simulink model "sampleModel1806"  (R2023a)
settings: Solver=VariableStepAuto  StartTime=0.0  StopTime=10.0  RelTol=1e-3
libraries: hdlsllib x4, simulink x1
settings Model: Creator=user1  LastModifiedBy=user1

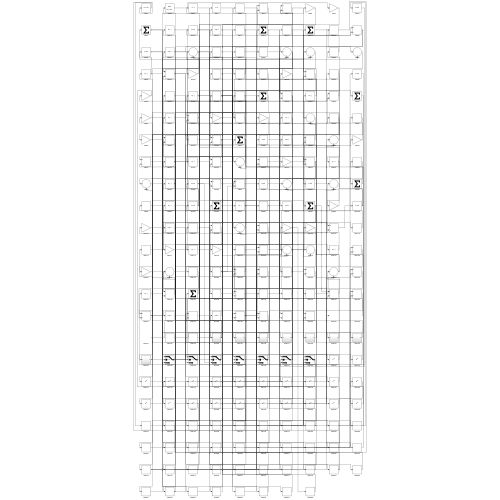
[thumbnail: Simulink's stored preview of the top-level diagram]
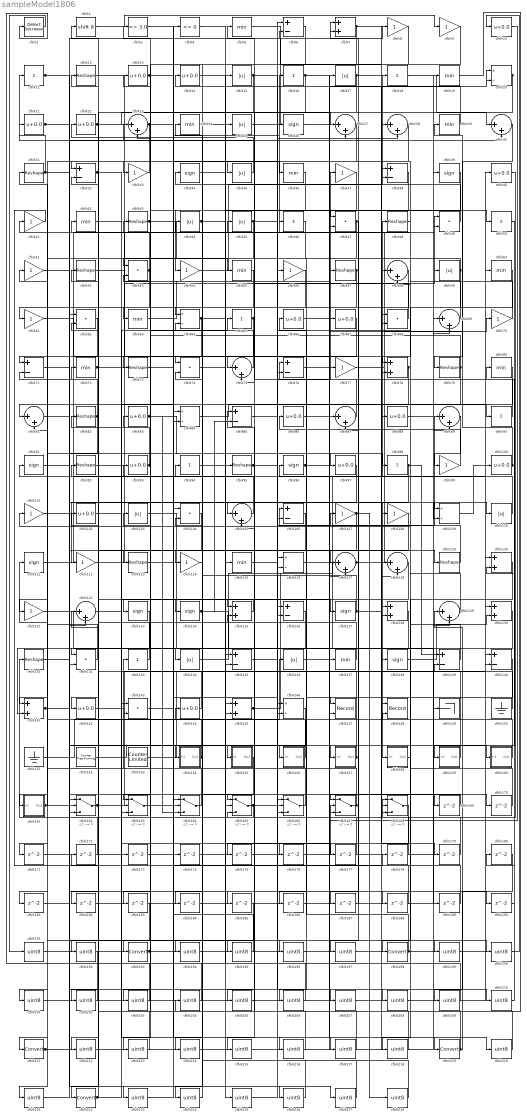
== system sampleModel1806 ==
  cfblk1 : simulink/Logic and Bit Operations/Detect Decrease  vinit=0.0  OutDataTypeStr=boolean
      settings: LibrarySourceBlock=|
      | hdlsllib/Logic and Bit
      | Operations/Detect
      | Decrease
  cfblk{10,13..14,21..22,40,66..67,83,86,88,93,97,100,102,142,144} (17 alike) : Bias  Bias=0.0  SaturateOnIntegerOverflow=off
  cfblk{8..9,33,37,41,51,54,56,61,70,77,99,101,107..108,112,114,121} (18 alike) : Gain
  cfblk{15,17,25,35,44..45,59,103,110,134,136} (11 alike) : Abs  SaturateOnIntegerOverflow=off
  cfblk{47,49,53,62,68,74,104,132,143} (9 alike) : DotProduct  OutDataTypeStr=Inherit: Inherit via internal rule
  cfblk{23,27..28,30,58,69,75,81,87,89,105,117..118,122,129} (15 alike) : Sum  Inputs=|++
  cfblk{6,32,38,71,76,85,106,126,135,139..140} (11 alike) : Sum  Inputs=+-
  cfblk{20,64,84,109,116,146} (6 alike) : Product  Inputs=*/  RndMeth=Zero  SaturateOnIntegerOverflow=on
  cfblk{11,16,18,46,50,65,90,94,98,133} (10 alike) : Sum  Inputs=+
  cfblk{26,34,39,91,96,111,123..124,127,138} (10 alike) : Signum
  cfblk{12,31,43,48,52,57,73,79,82,92,95,113,119,131} (14 alike) : Reshape
  cfblk{5,19,24,29,36,42,55,60,63,72,80,115,137} (13 alike) : MinMax
  cfblk{7,78,120,125,128,130,141,145} (8 alike) : Sum
  cfblk147 : Record  FileSettingsInternal="{\"entries\":[{\"content\":{\"excelSettings\":{\"content\":{},\"type\":\"Streamout.ExcelSettings\"}},\"type\":\"Streamout.FileSettingStorage\",\"uuid\":\"\"}],\"packageUris\":[\"http:\\/\\/schema.mathworks.com\\/mf0\\/streamout_blocks\\/R2020a\"],\"version\":\"1.0\"}"  Layout=[1 1]  SignalsInternal="{\"entries\":[{\"content\":{\"signals\":[{\"content\":{\"blockPath\":[],\"dimensions\":[1],\"domain\":\"\",\"lineColor\":\"#a2142f\",\"plots\":[1],\"port\":1,\"signalID\":4171,\"signalName\":\"XY Graph:1\"},\"type\":\"RecordBlkView.Signal\",\"uuid\":\"\"},{\"content\":{\"blockPath\":[],\"dimensions\":[1],\"domain\":\"\",\"lineColor\":\"#139fff\",\"plots\":[1],\"port\":2,\"signalID\":4174,\"signalName\":\"XY Graph:2\"},\"type\":\"RecordBlkView.Signal\",\"uuid\":\"\"}]},\"type\":\"RecordBlkView.InputSignals\",\"uuid\":\"\"}],\"packageUris\":[\"http:\\/\\/schema.mathworks.com\\/mf0\\/streamout_blocks\\/R2020a\"],\"version\":\"1.0\"}"  VisualizationBindings="{\"xyplotplugin\":{\"info\":[{\"series\":[{\"bindingParametersList\":[{\"parameter\":\"X-Axis\",\"signalID\":4171,\"signalName\":\"XY Graph:1\"},{\"parameter\":\"Y-Axis\",\"signalID\":4174,\"signalName\":\"XY Graph:2\"}],\"seriesID\":6691}],\"subplotID\":1}]}}"  CompatibilityTag=XY  st=-1
  cfblk148 : Record  FileSettingsInternal="{\"entries\":[{\"content\":{\"excelSettings\":{\"content\":{},\"type\":\"Streamout.ExcelSettings\"}},\"type\":\"Streamout.FileSettingStorage\",\"uuid\":\"\"}],\"packageUris\":[\"http:\\/\\/schema.mathworks.com\\/mf0\\/streamout_blocks\\/R2020a\"],\"version\":\"1.0\"}"  Layout=[1 1]  SignalsInternal="{\"entries\":[{\"content\":{\"signals\":[{\"content\":{\"blockPath\":[],\"dimensions\":[1],\"domain\":\"\",\"lineColor\":\"#a2142f\",\"plots\":[1],\"port\":1,\"signalID\":4179,\"signalName\":\"XY Graph:1\"},\"type\":\"RecordBlkView.Signal\",\"uuid\":\"\"},{\"content\":{\"blockPath\":[],\"dimensions\":[1],\"domain\":\"\",\"lineColor\":\"#139fff\",\"plots\":[1],\"port\":2,\"signalID\":4182,\"signalName\":\"XY Graph:2\"},\"type\":\"RecordBlkView.Signal\",\"uuid\":\"\"}]},\"type\":\"RecordBlkView.InputSignals\",\"uuid\":\"\"}],\"packageUris\":[\"http:\\/\\/schema.mathworks.com\\/mf0\\/streamout_blocks\\/R2020a\"],\"version\":\"1.0\"}"  VisualizationBindings="{\"xyplotplugin\":{\"info\":[{\"series\":[{\"bindingParametersList\":[{\"parameter\":\"X-Axis\",\"signalID\":4179,\"signalName\":\"XY Graph:1\"},{\"parameter\":\"Y-Axis\",\"signalID\":4182,\"signalName\":\"XY Graph:2\"}],\"seriesID\":17608}],\"subplotID\":1}]}}"  CompatibilityTag=XY  st=-1
  cfblk149 : Terminator
  cfblk150 : Ground
  cfblk151 : Ground
  cfblk152 : hdlsllib/Sources/Counter Free-Running  NumBits=16  tsamp=-1
  cfblk153 : hdlsllib/Sources/Counter Limited  uplimit=7  tsamp=-1
  cfblk154 : Subsystem
      settings: LibrarySourceBlock=|
      | hdlsllib/Ports &
      | Subsystems/Subsystem
  cfblk155 : Subsystem
      settings: LibrarySourceBlock=|
      | hdlsllib/Ports &
      | Subsystems/Subsystem
  cfblk156 : Subsystem
      settings: LibrarySourceBlock=|
      | hdlsllib/Ports &
      | Subsystems/Subsystem
  cfblk157 : Subsystem
      settings: LibrarySourceBlock=|
      | hdlsllib/Ports &
      | Subsystems/Subsystem
  cfblk158 : Subsystem
      settings: LibrarySourceBlock=|
      | hdlsllib/Ports &
      | Subsystems/Subsystem
  cfblk159 : Subsystem
      settings: LibrarySourceBlock=|
      | hdlsllib/Ports &
      | Subsystems/Subsystem
  cfblk160 : Subsystem
      settings: LibrarySourceBlock=|
      | hdlsllib/Ports &
      | Subsystems/Subsystem
  cfblk161 : Subsystem
      settings: LibrarySourceBlock=|
      | hdlsllib/Ports &
      | Subsystems/Subsystem
  cfblk{162..168} (7 alike) : Switch  SaturateOnIntegerOverflow=off  InputSameDT=off
  cfblk{169..190} (22 alike) : Delay  SampleTime=1
  cfblk{191..192,194..197,199..210,212..218,220..221,223..228} (33 alike) : DataTypeConversion  OutDataTypeStr=uint8  SaturateOnIntegerOverflow=off  RndMeth=Floor
  cfblk{193,198,211,219,222} (5 alike) : DataTypeConversion  SaturateOnIntegerOverflow=off  RndMeth=Floor
  cfblk2 : ArithShift  BitShiftNumber=8
  cfblk3 : hdlsllib/Logic and Bit Operations/Compare To Constant  relop=<=  const=3.0  OutDataTypeStr=boolean
  cfblk4 : hdlsllib/Logic and Bit Operations/Compare To Zero  relop=<=  OutDataTypeStr=boolean
  wires:
  cfblk38/1 -> cfblk54/1
  cfblk45/1 -> cfblk61/1, cfblk210/1
  cfblk165/1 -> cfblk131/1, cfblk28/2
  cfblk84/1 -> cfblk90/1
  cfblk2/1 -> cfblk9/1
  cfblk139/1 -> cfblk101/1
  cfblk52/1 -> cfblk74/1
  cfblk50/1 -> cfblk159/1(In1)
  cfblk121/1 -> cfblk134/1
  cfblk48/1 -> cfblk35/1
  cfblk161/1(Out1) -> cfblk111/1, cfblk190/1
  cfblk69/1 -> cfblk49/1
  cfblk82/1 -> cfblk141/1, cfblk71/2
  cfblk111/1 -> cfblk49/2
  cfblk117/1 -> cfblk70/1, cfblk179/1
  cfblk104/1 -> cfblk222/1
  cfblk12/1 -> cfblk75/1
  cfblk164/1 -> cfblk133/1
  cfblk76/1 -> cfblk37/1
  cfblk98/1 -> cfblk158/1(In1), cfblk139/1, cfblk147/1
  cfblk129/1 -> cfblk86/1, cfblk34/1
  cfblk97/1 -> cfblk112/1
  cfblk47/1 -> cfblk186/1, cfblk187/1, cfblk202/1
  cfblk73/1 -> cfblk97/1
  cfblk132/1 -> cfblk91/1
  cfblk146/1 -> cfblk162/2
  cfblk25/1 -> cfblk8/1
  cfblk54/1 -> cfblk18/1
  cfblk99/1 -> cfblk66/1
  cfblk33/1 -> cfblk32/1
  cfblk43/1 -> cfblk115/1, cfblk26/1
  cfblk109/1 -> cfblk100/1
  cfblk141/1 -> cfblk6/2, cfblk223/1
  cfblk153/1 -> cfblk15/1
  cfblk4/1 -> cfblk95/1
  cfblk22/1 -> cfblk55/1, cfblk27/1
  cfblk57/1 -> cfblk132/1, cfblk135/2
  cfblk163/1 -> cfblk4/1
  cfblk134/1 -> cfblk48/1
  cfblk159/1(Out1) -> cfblk82/1
  cfblk53/1 -> cfblk43/1, cfblk71/1
  cfblk123/1 -> cfblk141/2
  cfblk112/1 -> cfblk59/1
  cfblk115/1 -> cfblk107/1
  cfblk75/1 -> cfblk3/1
  cfblk152/1 -> cfblk157/1(In1)
  cfblk133/1 -> cfblk32/2
  cfblk77/1 -> cfblk39/1
  cfblk78/1 -> cfblk105/2, cfblk182/1
  cfblk6/1 -> cfblk154/1(In1)
  cfblk119/1 -> cfblk106/1
  cfblk157/1(Out1) -> cfblk42/1, cfblk144/1
  cfblk56/1 -> cfblk211/1
  cfblk34/1 -> cfblk47/1
  cfblk14/1 -> cfblk119/1
  cfblk29/1 -> cfblk14/1
  cfblk145/1 -> cfblk89/1, cfblk139/2, cfblk85/1
  cfblk63/1 -> cfblk25/1
  cfblk95/1 -> cfblk77/1, cfblk169/1
  cfblk70/1 -> cfblk41/1
  cfblk46/1 -> cfblk81/1
  cfblk31/1 -> cfblk11/1, cfblk98/1
  cfblk167/1 -> cfblk7/1, cfblk51/1
  cfblk122/1 -> cfblk219/1
  cfblk80/1 -> cfblk161/1(In1)
  cfblk65/1 -> cfblk155/1(In1), cfblk113/1
  cfblk92/1 -> cfblk57/1
  cfblk20/1 -> cfblk75/2, cfblk165/2
  cfblk116/1 -> cfblk138/1
  cfblk32/1 -> cfblk105/1, cfblk177/1
  cfblk110/1 -> cfblk76/1
  cfblk40/1 -> cfblk168/1
  cfblk68/1 -> cfblk45/1
  cfblk18/1 -> cfblk30/1
  cfblk103/1 -> cfblk148/1
  cfblk35/1 -> cfblk22/1
  cfblk7/1 -> cfblk88/1, cfblk224/1
  cfblk72/1 -> cfblk16/1, cfblk125/1
  cfblk101/1 -> cfblk60/1
  cfblk160/1(Out1) -> cfblk2/1
  cfblk142/1 -> cfblk130/1
  cfblk150/1 -> cfblk68/1
  cfblk137/1 -> cfblk23/2
  cfblk10/1 -> cfblk167/2
  cfblk151/1 -> cfblk136/1
  cfblk51/1 -> cfblk164/2
  cfblk107/1 -> cfblk163/3, cfblk228/1
  cfblk79/1 -> cfblk117/1, cfblk53/2, cfblk181/1
  cfblk162/1 -> cfblk87/1, cfblk65/1, cfblk165/1
  cfblk55/1 -> cfblk163/1
  cfblk93/1 -> cfblk72/1, cfblk83/1
  cfblk125/1 -> cfblk124/1
  cfblk59/1 -> cfblk53/1, cfblk106/2, cfblk194/1, cfblk197/1
  cfblk85/1 -> cfblk76/2
  cfblk124/1 -> cfblk127/1, cfblk85/2, cfblk189/1
  cfblk154/1(Out1) -> cfblk12/1, cfblk31/1
  cfblk13/1 -> cfblk176/1, cfblk217/1
  cfblk136/1 -> cfblk17/1
  cfblk135/1 -> cfblk68/2
  cfblk144/1 -> cfblk103/1
  cfblk49/1 -> cfblk5/1
  cfblk127/1 -> cfblk20/1, cfblk64/2
  cfblk87/1 -> cfblk21/1
  cfblk5/1 -> cfblk58/1
  cfblk100/1 -> cfblk67/1, cfblk29/1
  cfblk17/1 -> cfblk38/1, cfblk47/2
  cfblk16/1 -> cfblk50/1, cfblk142/1
  cfblk138/1 -> cfblk130/2
  cfblk21/1 -> cfblk110/1, cfblk160/1(In1)
  cfblk158/1(Out1) -> cfblk38/2
  cfblk58/1 -> cfblk121/1
  cfblk37/1 -> cfblk123/1
  cfblk15/1 -> cfblk63/1, cfblk78/2
  cfblk44/1 -> cfblk109/1, cfblk188/1, cfblk199/1, cfblk200/1
  cfblk166/1 -> cfblk102/1
  cfblk156/1(Out1) -> cfblk93/1
  cfblk11/1 -> cfblk118/1, cfblk163/2
  cfblk61/1 -> cfblk118/2
  cfblk3/1 -> cfblk36/1
  cfblk36/1 -> cfblk64/1
  cfblk88/1 -> cfblk69/2
  cfblk23/1 -> cfblk132/2, cfblk146/2, cfblk109/2
  cfblk105/1 -> cfblk81/2
  cfblk30/1 -> cfblk79/1
  cfblk90/1 -> cfblk44/1
  cfblk91/1 -> cfblk28/1
  cfblk60/1 -> cfblk78/1
  cfblk86/1 -> cfblk137/1
  cfblk8/1 -> cfblk33/1
  cfblk120/1 -> cfblk198/1
  cfblk108/1 -> cfblk193/1
  cfblk89/1 -> cfblk99/1
  cfblk83/1 -> cfblk166/3, cfblk164/3
  cfblk27/1 -> cfblk114/1, cfblk116/2, cfblk147/2
  cfblk96/1 -> cfblk156/1(In1), cfblk20/2
  cfblk130/1 -> cfblk145/2
  cfblk42/1 -> cfblk84/2
  cfblk74/1 -> cfblk46/1
  cfblk64/1 -> cfblk73/1, cfblk30/2
  cfblk169/1 -> cfblk167/1
  cfblk102/1 -> cfblk170/1
  cfblk170/1 -> cfblk58/2
  cfblk28/1 -> cfblk171/1
  cfblk171/1 -> cfblk145/1
  cfblk172/1 -> cfblk162/1
  cfblk173/1 -> cfblk27/2
  cfblk174/1 -> cfblk167/3
  cfblk168/1 -> cfblk175/1
  cfblk175/1 -> cfblk116/1
  cfblk176/1 -> cfblk89/2
  cfblk177/1 -> cfblk23/1
  cfblk41/1 -> cfblk178/1
  cfblk178/1 -> cfblk146/1
  cfblk179/1 -> cfblk87/2
  cfblk181/1 -> cfblk162/3
  cfblk182/1 -> cfblk6/1
  cfblk9/1 -> cfblk183/1
  cfblk155/1(Out1) -> cfblk184/1
  cfblk184/1 -> cfblk69/1
  cfblk113/1 -> cfblk185/1
  cfblk186/1 -> cfblk129/2
  cfblk187/1 -> cfblk7/2
  cfblk188/1 -> cfblk84/1
  cfblk189/1 -> cfblk125/2
  cfblk190/1 -> cfblk80/1
  cfblk1/1 -> cfblk191/1
  cfblk191/1 -> cfblk10/1
  cfblk183/1 -> cfblk192/1
  cfblk192/1 -> cfblk1/1
  cfblk193/1 -> cfblk174/1, cfblk168/2
  cfblk194/1 -> cfblk108/1
  cfblk128/1 -> cfblk195/1
  cfblk195/1 -> cfblk164/1
  cfblk71/1 -> cfblk196/1
  cfblk196/1 -> cfblk128/1
  cfblk197/1 -> cfblk128/2
  cfblk198/1 -> cfblk148/2, cfblk96/1, cfblk218/1
  cfblk199/1 -> cfblk120/1
  cfblk200/1 -> cfblk120/2
  cfblk62/1 -> cfblk201/1
  cfblk201/1 -> cfblk40/1
  cfblk202/1 -> cfblk62/1
  cfblk67/1 -> cfblk203/1
  cfblk203/1 -> cfblk62/2
  cfblk19/1 -> cfblk204/1
  cfblk204/1 -> cfblk92/1
  cfblk106/1 -> cfblk205/1
  cfblk205/1 -> cfblk19/1
  cfblk140/1 -> cfblk206/1
  cfblk206/1 -> cfblk13/1
  cfblk131/1 -> cfblk207/1
  cfblk207/1 -> cfblk140/1
  cfblk26/1 -> cfblk208/1
  cfblk208/1 -> cfblk140/2
  cfblk180/1 -> cfblk209/1
  cfblk209/1 -> cfblk135/1
  cfblk210/1 -> cfblk180/1
  cfblk211/1 -> cfblk117/2, cfblk168/3, cfblk149/1
  cfblk118/1 -> cfblk212/1
  cfblk212/1 -> cfblk56/1
  cfblk126/1 -> cfblk213/1
  cfblk213/1 -> cfblk52/1
  cfblk114/1 -> cfblk214/1
  cfblk214/1 -> cfblk126/1
  cfblk39/1 -> cfblk215/1
  cfblk215/1 -> cfblk126/2
  cfblk143/1 -> cfblk216/1
  cfblk216/1 -> cfblk74/2
  cfblk217/1 -> cfblk143/1
  cfblk218/1 -> cfblk143/2
  cfblk219/1 -> cfblk165/3, cfblk129/1
  cfblk66/1 -> cfblk220/1
  cfblk220/1 -> cfblk122/1
  cfblk185/1 -> cfblk221/1
  cfblk221/1 -> cfblk122/2
  cfblk222/1 -> cfblk173/1, cfblk172/1
  cfblk223/1 -> cfblk104/1
  cfblk224/1 -> cfblk104/2
  cfblk94/1 -> cfblk225/1
  cfblk225/1 -> cfblk166/2
  cfblk81/1 -> cfblk226/1
  cfblk226/1 -> cfblk94/1
  cfblk24/1 -> cfblk227/1
  cfblk227/1 -> cfblk166/1
  cfblk228/1 -> cfblk24/1

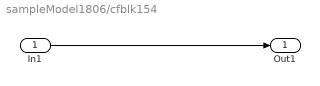
== system sampleModel1806/cfblk154 ==
  In1 : Inport
  Out1 : Outport
  wires:
  In1/1 -> Out1/1

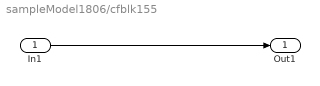
== system sampleModel1806/cfblk155 ==
  In1 : Inport
  Out1 : Outport
  wires:
  In1/1 -> Out1/1

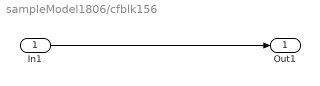
== system sampleModel1806/cfblk156 ==
  In1 : Inport
  Out1 : Outport
  wires:
  In1/1 -> Out1/1

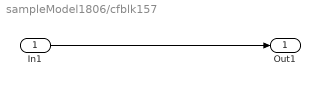
== system sampleModel1806/cfblk157 ==
  In1 : Inport
  Out1 : Outport
  wires:
  In1/1 -> Out1/1

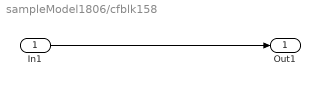
== system sampleModel1806/cfblk158 ==
  In1 : Inport
  Out1 : Outport
  wires:
  In1/1 -> Out1/1

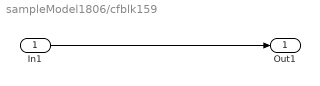
== system sampleModel1806/cfblk159 ==
  In1 : Inport
  Out1 : Outport
  wires:
  In1/1 -> Out1/1

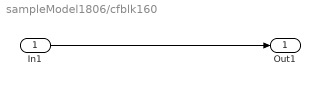
== system sampleModel1806/cfblk160 ==
  In1 : Inport
  Out1 : Outport
  wires:
  In1/1 -> Out1/1

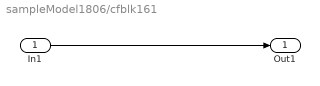
== system sampleModel1806/cfblk161 ==
  In1 : Inport
  Out1 : Outport
  wires:
  In1/1 -> Out1/1
